simulink subsystem "NoDifferentialControl"  (R2024a)
settings: Solver=VariableStepAuto  StartTime=0.0  StopTime=10.0  RelTol=1e-3
settings Model: Creator=The MathWorks, Inc.  LastModifiedBy=The MathWorks, Inc.
settings RTWCC: GPUComputeCapability=3.5

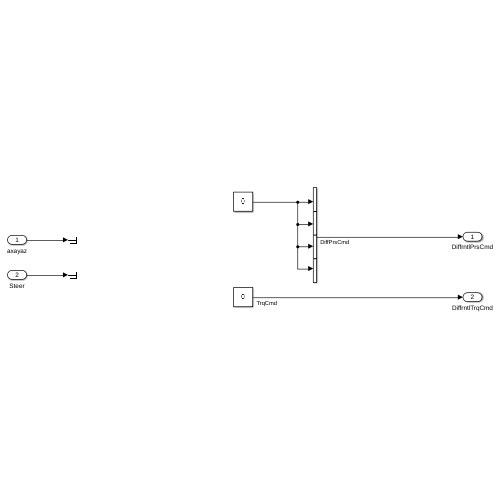
[thumbnail: Simulink's stored preview of the top-level diagram]
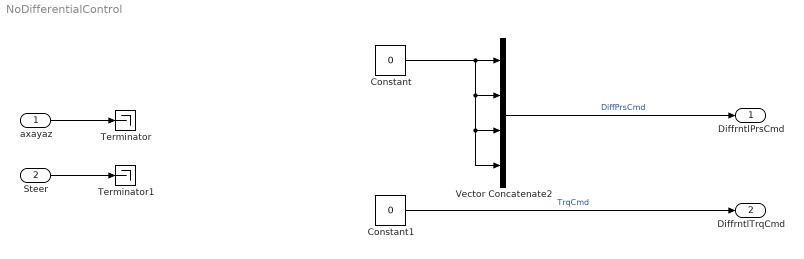
== system NoDifferentialControl ==
  axayaz : Inport
  Steer : Inport  Port=2
  Constant : Constant  Value=0  SampleTime=10/1000
  Constant1 : Constant  Value=0  SampleTime=10/1000
  Terminator : Terminator
  Terminator1 : Terminator
  Vector Concatenate2 : Concatenate  NumInputs=4
  DiffrntlPrsCmd : Outport  VectorParamsAs1DForOutWhenUnconnected=off
  DiffrntlTrqCmd : Outport  Port=2  VectorParamsAs1DForOutWhenUnconnected=off
  wires:
  Constant/1 -> Vector Concatenate2/2, Vector Concatenate2/3, Vector Concatenate2/4, Vector Concatenate2/1
  Steer/1 -> Terminator1/1
  Vector Concatenate2/1 -> DiffrntlPrsCmd/1  "DiffPrsCmd"
  axayaz/1 -> Terminator/1
  Constant1/1 -> DiffrntlTrqCmd/1  "TrqCmd"
